simulink model "Janina_hobe_kina_v1"  (R2018a)
settings: Solver=VariableStepAuto  StartTime=0.0  StopTime=0.5  RelTol=1e-3
libraries: fl_lib x37, nesl_utility x19, elec_lib x10, pe_lib x4, powerlib_meascontrol x4
settings Model: Creator=ASUS  LastModifiedBy=ASUS
settings SolverCC: ZeroCrossAlgorithm=Adaptive
settings DebuggingCC: MaxConsecutiveZCsMsg=none

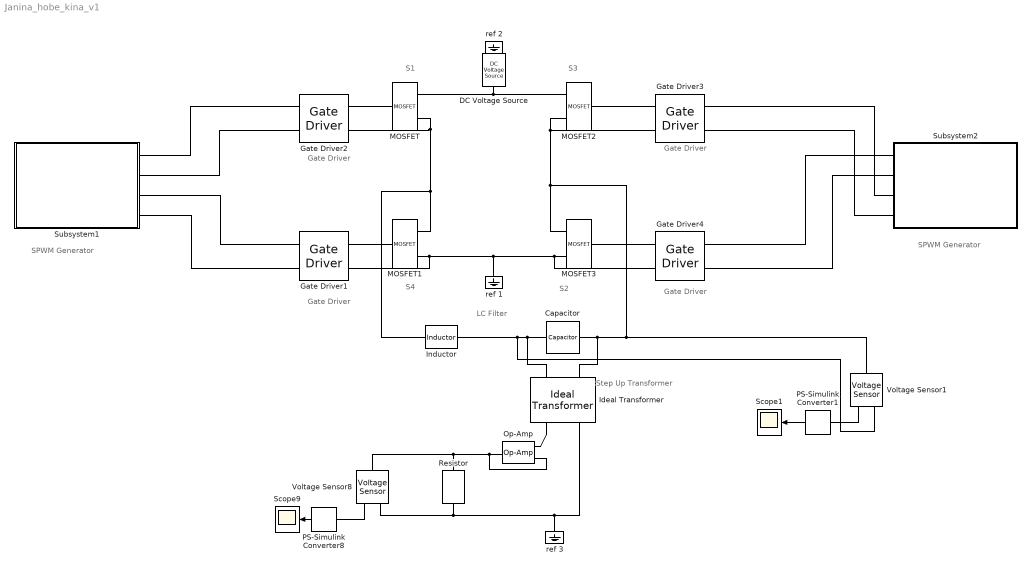
== system Janina_hobe_kina_v1 ==
  note: LC Filter
  note: S1
  note: Gate Driver
  note: SPWM Generator
  note: SPWM Generator
  note: Gate Driver
  note: Gate Driver
  note: Gate Driver
  note: S2
  note: S3
  note: S4
  note: Step Up Transformer
  Capacitor : fl_lib/Electrical/Electrical Elements/Capacitor  c=47e-6 F  r=1e-6 Ohm  g=0 1/Ohm  i_specify=off  i_priority=None  i=0 A  i_nominal_specify=off  i_nominal_unit=A  i_nominal_value=1  v_specify=off  v_priority=None  v=0 V  v_nominal_specify=off  v_nominal_unit=V  v_nominal_value=1  vc_specify=off  vc_priority=High  vc=0 V  vc_nominal_specify=off  vc_nominal_unit=V  vc_nominal_value=1
  DC Voltage Source : fl_lib/Electrical/Electrical Sources/DC Voltage Source  v0=12 V
  Gate Driver{1..4} (4 alike) : elec_lib/Actuators & Drivers/Drivers/Gate Driver  vHigh=15 V  vLow=0 V  parameterization=1  rHigh=2 Ohm  rLow=2 Ohm  tRise=20 ns  tFall=20 ns  cLoad=10 nF  enable_faults=0  t_fault=1 s  fault_type=1  uHighValue=0.7  uLowValue=0.3  tHigh=50 ns  tLow=50 ns  ZonTime_specify=off  ZonTime_priority=None  ZonTime=0 s  ZoffTime_specify=off  ZoffTime_priority=None  ZoffTime=0 s  uHigh=2.0 V  uLow=0.8 V
      settings: SourceProductName=Simscape Electronics  SourceProductBaseCode=SN
  Ideal Transformer : fl_lib/Electrical/Electrical Elements/Ideal Transformer  n=12/220  i1_specify=off  i1_priority=None  i1=0 A  i1_nominal_specify=off  i1_nominal_unit=A  i1_nominal_value=1  v1_specify=off  v1_priority=None  v1=0 V  v1_nominal_specify=off  v1_nominal_unit=V  v1_nominal_value=1  i2_specify=off  i2_priority=None  i2=0 A  i2_nominal_specify=off  i2_nominal_unit=A  i2_nominal_value=1  v2_specify=off  v2_priority=None  v2=0 V  v2_nominal_specify=off  v2_nominal_unit=V  v2_nominal_value=1
      settings: SourceProductName=Simscape  SourceProductBaseCode=SS
  Inductor : elec_lib/Passive Devices/Inductor  l=0.46 H  L_tol=20  enable_L_tol=0  tol_distribution=1  nSigma=4  r=0 Ohm  g=1e-9 1/Ohm  enable_operating_limits=0  operating_limit_action=2  max_working_current=1 A  power_rating=1 W  enable_faults=0  fault_action=1  lambdaPercent=50  k_faulted=0.9999  turnsShort=0  openCct=0  groundShort=0  groundShortG=0 1/Ohm  tau_fault=1e-3 s  enable_temporal_fault=0  t_fault=1 s  enable_behavioral_fault=0  max_permissible_voltage=100 V  n_fail_on_voltage=1  max_permissible_current=1 A  t_fail_on_current=1 s  i_L_specify=off  i_L_priority=High  i_L=0 A  i_L_nominal_specify=off  i_L_nominal_unit=A  i_L_nominal_value=1
      settings: SourceProductName=Simscape Electronics  SourceProductBaseCode=SN
  MOSFET{,1..3} (4 alike) : pe_lib/Semiconductors/Fundamental Components/MOSFET  Rds=0.01 Ohm  Goff=1e-6 1/Ohm  Vth=2 V  diode_param=2  diode_Vf=0.8 V  diode_Ron=0.001 Ohm  diode_Goff=1e-5 1/Ohm  diode_C=5e-8 F  diode_iRM=-235 A  diode_iF=300 A  diode_idot=-50 A/us  diode_trr_param=1  diode_trr_factor=3  diode_trr=15 us  diode_Qrr=1.5e+3 s*uA  thermal_loss_option=2  Voff=300 V  Tau=1e-4 s  Tj=[ 298.15 398.15 ] K  Iout_scalar=600 A  Eon_scalar=0.02286 J  Eoff_scalar=0.01714 J  Von_scalar=2.7 V  Iout_data=[ 0 10 50 100 200 400 600 ] A  Eon_data=[ 0 2.9e-4 0.00143 0.00286 0.00571 0.01314 0.02286; 0 5.7e-4 0.00263 0.00514 0.01029 0.02057 0.03029 ] J  Eoff_data=[ 0 2.1e-4 0.00107 0.00214 0.00429 0.009859999999999999 0.01714; 0 4.3e-4 0.00197 0.00386 0.00771 0.01543 0.02271 ] J  Von_data=[ 0 1.1 1.3 1.45 1.75 2.25 2.7; 0 1 1.15 1.35 1.7 2.35 3 ] V
      settings: SourceProductName=Simscape Power Systems  SourceProductBaseCode=PS
  Op-Amp : fl_lib/Electrical/Electrical Elements/Op-Amp  outI_specify=off  outI_priority=None  outI=0 A  outI_nominal_specify=off  outI_nominal_unit=A  outI_nominal_value=1
  PS-Simulink Converter1 : nesl_utility/PS-Simulink Converter  PhysicalDomain=network_engine_domain  SubClassName=ps_output  LeftPortType=input  RightPortType=output  PseudoPeriodic=off  Frequencies=[]  Unit=1  AffineConversion=off
  PS-Simulink Converter8 : nesl_utility/PS-Simulink Converter  PhysicalDomain=network_engine_domain  SubClassName=ps_output  LeftPortType=input  RightPortType=output  PseudoPeriodic=off  Frequencies=[]  Unit=1  AffineConversion=off
  Resistor : elec_lib/Passive Devices/Resistor  R=100 Ohm  R_tol=5  enable_R_tol=0  tol_distribution=1  nSigma=4  enable_operating_limits=0  operating_limit_action=2  max_working_voltage=100 V  power_rating=1 W  enable_faults=0  fault_action=1  R_faulted=inf Ohm  enable_temporal_fault=0  t_fault=1 s  enable_behavioral_fault=0  max_permissible_current=1 A  t_fail_on_current=1 s  noise_mode=0  sample_time=1e-3 s  repeatability=1  auto_seed=3626636697  user_seed=0  Tdevice=25 degC  alpha=3.93e-3 1/K  Tmeas=25 degC  thermal_mass=100 J/K  power_derating_T1=70 degC  power_derating_T2=155 degC  operating_temperature_range_vec=[-50, 150] degC  temperature_specify=off  temperature_priority=High  temperature=298.15 K  temperature_nominal_specify=off  temperature_nominal_unit=K  temperature_nominal_value=1
  Scope1 : Scope
  Scope9 : Scope
  Subsystem1 : Subsystem
  Subsystem2 : Subsystem
  Voltage Sensor1 : fl_lib/Electrical/Electrical Sensors/Voltage Sensor
  Voltage Sensor8 : fl_lib/Electrical/Electrical Sensors/Voltage Sensor
  ref 1 : fl_lib/Electrical/Electrical Elements/Electrical Reference
  ref 2 : fl_lib/Electrical/Electrical Elements/Electrical Reference
  ref 3 : fl_lib/Electrical/Electrical Elements/Electrical Reference
  wires:
  PS-Simulink Converter8/1 -> Scope9/1
  PS-Simulink Converter1/1 -> Scope1/1
  connections:
  MOSFET/RConn2 -- Gate Driver2/RConn2 -- Inductor/LConn1 -- MOSFET1/RConn1
  ref 2/LConn1 -- DC Voltage Source/RConn1
  MOSFET/RConn1 -- MOSFET2/RConn1 -- DC Voltage Source/LConn1
  MOSFET3/RConn2 -- Gate Driver4/RConn2 -- ref 1/LConn1 -- Gate Driver1/RConn2 -- MOSFET1/RConn2
  Subsystem1/RConn4 -- Gate Driver1/LConn2
  Gate Driver2/LConn1 -- Subsystem1/RConn1
  Gate Driver2/LConn2 -- Subsystem1/RConn2
  Gate Driver1/LConn1 -- Subsystem1/RConn3
  Subsystem2/RConn1 -- Gate Driver4/LConn1
  Subsystem2/RConn2 -- Gate Driver4/LConn2
  Gate Driver3/LConn1 -- Subsystem2/RConn3
  Gate Driver3/LConn2 -- Subsystem2/RConn4
  Gate Driver3/RConn1 -- MOSFET2/LConn1
  Gate Driver4/RConn1 -- MOSFET3/LConn1
  Gate Driver2/RConn1 -- MOSFET/LConn1
  Gate Driver1/RConn1 -- MOSFET1/LConn1
  Capacitor/LConn1 -- Ideal Transformer/LConn1 -- Voltage Sensor1/RConn2 -- Inductor/RConn1
  Op-Amp/LConn1 -- Voltage Sensor8/LConn1 -- Resistor/LConn1 -- Op-Amp/RConn1
  Ideal Transformer/RConn1 -- Op-Amp/LConn2
  Resistor/RConn1 -- ref 3/LConn1 -- Ideal Transformer/RConn2 -- Voltage Sensor8/RConn2
  Voltage Sensor8/RConn1 -- PS-Simulink Converter8/LConn1
  Capacitor/RConn1 -- Voltage Sensor1/LConn1 -- MOSFET3/RConn1 -- Gate Driver3/RConn2 -- MOSFET2/RConn2 -- Ideal Transformer/LConn2
  Voltage Sensor1/RConn1 -- PS-Simulink Converter1/LConn1

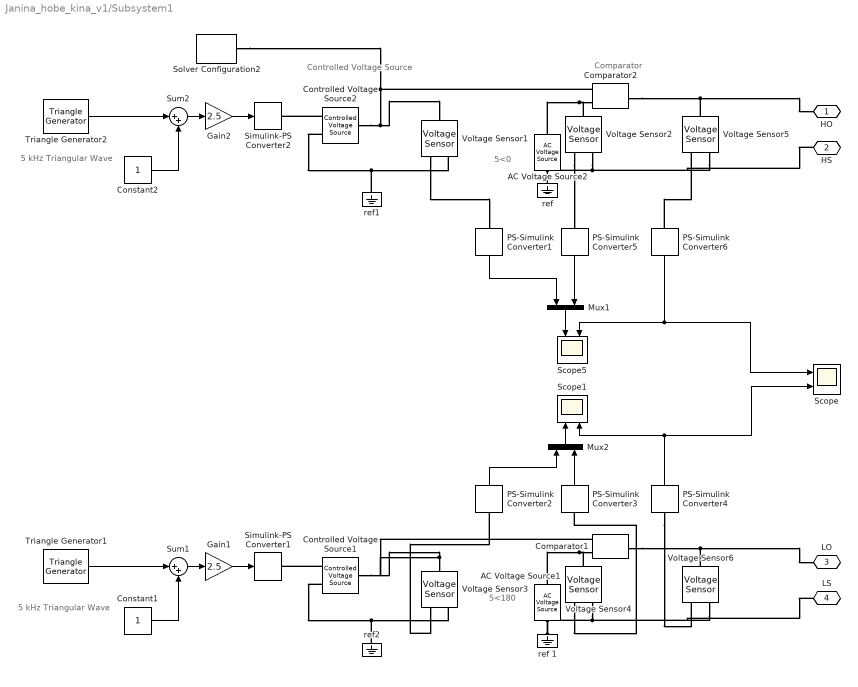
== system Janina_hobe_kina_v1/Subsystem1 ==
  note: Controlled Voltage Source
  note: Comparator
  note: 5 kHz
      | Triangular Wave
  note: 5<180
  note: 5<0
  note: 5 kHz
      | Triangular Wave
  AC Voltage Source1 : fl_lib/Electrical/Electrical Sources/AC Voltage Source  amp=5 V  shift=180 deg  frequency=50 Hz  omega=0 rad/s
  AC Voltage Source2 : fl_lib/Electrical/Electrical Sources/AC Voltage Source  amp=5 V  shift=0 deg  frequency=50 Hz  omega=0 rad/s
  Comparator1 : elec_lib/Integrated Circuits/Comparator  V_OS=5 mV  V_OL=0 V  V_OH=5 V  C_IN=0 pF  R_OUT=50 Ohm  Delay=0 s
      settings: SourceProductName=Simscape Electronics  SourceProductBaseCode=SN
  Comparator2 : elec_lib/Integrated Circuits/Comparator  V_OS=5 mV  V_OL=0 V  V_OH=5 V  C_IN=0 pF  R_OUT=50 Ohm  Delay=0 s
      settings: SourceProductName=Simscape Electronics  SourceProductBaseCode=SN
  Constant1 : Constant
  Constant2 : Constant
  Controlled Voltage Source1 : fl_lib/Electrical/Electrical Sources/Controlled Voltage Source
  Controlled Voltage Source2 : fl_lib/Electrical/Electrical Sources/Controlled Voltage Source
  Gain1 : Gain  Gain=2.5
  Gain2 : Gain  Gain=2.5
  Mux1 : Mux  Inputs=2
  Mux2 : Mux  Inputs=2
  PS-Simulink Converter{1..6} (6 alike) : nesl_utility/PS-Simulink Converter  PhysicalDomain=network_engine_domain  SubClassName=ps_output  LeftPortType=input  RightPortType=output  PseudoPeriodic=off  Frequencies=[]  Unit=1  AffineConversion=off
  Scope : Scope  NumInputPorts=2
  Scope1 : Scope  NumInputPorts=2
  Scope5 : Scope  NumInputPorts=2
  Simulink-PS Converter1 : nesl_utility/Simulink-PS Converter  PhysicalDomain=network_engine_domain  SubClassName=ps_input  LeftPortType=input  RightPortType=output  PseudoPeriodic=off  Frequencies=[]  NoiseDistribution=none  NoiseParameters=[]  Unit=1  AffineConversion=off  FilteringAndDerivatives=provide  SimscapeFilterOrder=1  InputFilterTimeConstant=0.001  UdotUserProvided=0
  Simulink-PS Converter2 : nesl_utility/Simulink-PS Converter  PhysicalDomain=network_engine_domain  SubClassName=ps_input  LeftPortType=input  RightPortType=output  PseudoPeriodic=off  Frequencies=[]  NoiseDistribution=none  NoiseParameters=[]  Unit=1  AffineConversion=off  FilteringAndDerivatives=provide  SimscapeFilterOrder=1  InputFilterTimeConstant=0.001  UdotUserProvided=0
  Solver Configuration2 : nesl_utility/Solver Configuration  PhysicalDomain=network_engine_domain  SubClassName=solver  LeftPortType=input  RightPortType=generic  Tones=[]  Harmonics=[]  SimulateNoise=off  Profile=off  UseLocalSampling=off  EnableSwitchedLinearOptims=on  FrequencyDomain=off  UseCCode=off  RelTol=0.001  AbsTol=1e-06  MinStep=1e-09  ToWorkspace=off  RevertToSquareIcSolve=off  NumHomotopyIterations=100  PhasorMode=off  PhasorModeNumHarmonics=1  DoDC=off  ResidualTolerance=1e-09  UseLocalSolver=off  LocalSolverChoice=NE_BACKWARD_EULER_ADVANCER  LocalSolverSampleTime=0.001  DoFixedCost=off  MaxNonlinIter=3  MaxModeIter=2  LinearAlgebra=Sparse  EquationFormulation=NE_TIME_EF  DelaysMemoryBudget=1024  AutomaticFiltering=on  FilteringTimeConstant=0.001
  Sum1 : Sum  Inputs=|++
  Sum2 : Sum  Inputs=|++
  Triangle Generator1 : powerlib_meascontrol/Pulse & Signal Generators/Triangle Generator  Freq=5e3  Phase=0  Ts=0
  Triangle Generator2 : powerlib_meascontrol/Pulse & Signal Generators/Triangle Generator  Freq=5e3  Phase=0  Ts=0
  Voltage Sensor{1..6} (6 alike) : fl_lib/Electrical/Electrical Sensors/Voltage Sensor
  "ref " : fl_lib/Electrical/Electrical Elements/Electrical Reference
  ref 1 : fl_lib/Electrical/Electrical Elements/Electrical Reference
  ref1 : fl_lib/Electrical/Electrical Elements/Electrical Reference
  ref2 : fl_lib/Electrical/Electrical Elements/Electrical Reference
  HO : PMIOPort  Side=Right
  HS : PMIOPort  Port=2  Side=Right
  LO : PMIOPort  Port=3  Side=Right
  LS : PMIOPort  Port=4  Side=Right
  wires:
  Triangle Generator2/1 -> Sum2/1
  Sum2/1 -> Gain2/1
  Constant2/1 -> Sum2/2
  Gain2/1 -> Simulink-PS Converter2/1
  PS-Simulink Converter5/1 -> Mux1/2
  PS-Simulink Converter1/1 -> Mux1/1
  Mux1/1 -> Scope5/1
  PS-Simulink Converter6/1 -> Scope/1, Scope5/2
  Constant1/1 -> Sum1/2
  Sum1/1 -> Gain1/1
  Gain1/1 -> Simulink-PS Converter1/1
  Triangle Generator1/1 -> Sum1/1
  PS-Simulink Converter2/1 -> Mux2/1
  PS-Simulink Converter3/1 -> Mux2/2
  Mux2/1 -> Scope1/1
  PS-Simulink Converter4/1 -> Scope/2, Scope1/2
  connections:
  Solver Configuration2/RConn1 -- Controlled Voltage Source2/LConn1 -- Voltage Sensor1/LConn1 -- Comparator2/LConn2
  Comparator2/RConn1 -- Voltage Sensor5/LConn1 -- HO/RConn1
  Controlled Voltage Source2/RConn1 -- Simulink-PS Converter2/RConn1
  ref1/LConn1 -- Voltage Sensor1/RConn2 -- Controlled Voltage Source2/RConn2
  Voltage Sensor1/RConn1 -- PS-Simulink Converter1/LConn1
  "ref "/LConn1 -- Voltage Sensor5/RConn2 -- HS/RConn1 -- Voltage Sensor2/RConn2 -- AC Voltage Source2/RConn1
  AC Voltage Source2/LConn1 -- Voltage Sensor2/LConn1 -- Comparator2/LConn1
  Voltage Sensor2/RConn1 -- PS-Simulink Converter5/LConn1
  PS-Simulink Converter6/LConn1 -- Voltage Sensor5/RConn1
  Comparator1/RConn1 -- Voltage Sensor6/LConn1 -- LO/RConn1
  Voltage Sensor3/LConn1 -- Comparator1/LConn2 -- Controlled Voltage Source1/LConn1
  Controlled Voltage Source1/RConn2 -- ref2/LConn1 -- Voltage Sensor3/RConn2
  AC Voltage Source1/RConn1 -- ref 1/LConn1 -- Voltage Sensor6/RConn2 -- LS/RConn1 -- Voltage Sensor4/RConn2
  AC Voltage Source1/LConn1 -- Voltage Sensor4/LConn1 -- Comparator1/LConn1
  Controlled Voltage Source1/RConn1 -- Simulink-PS Converter1/RConn1
  Voltage Sensor3/RConn1 -- PS-Simulink Converter2/LConn1
  PS-Simulink Converter4/LConn1 -- Voltage Sensor6/RConn1
  Voltage Sensor4/RConn1 -- PS-Simulink Converter3/LConn1

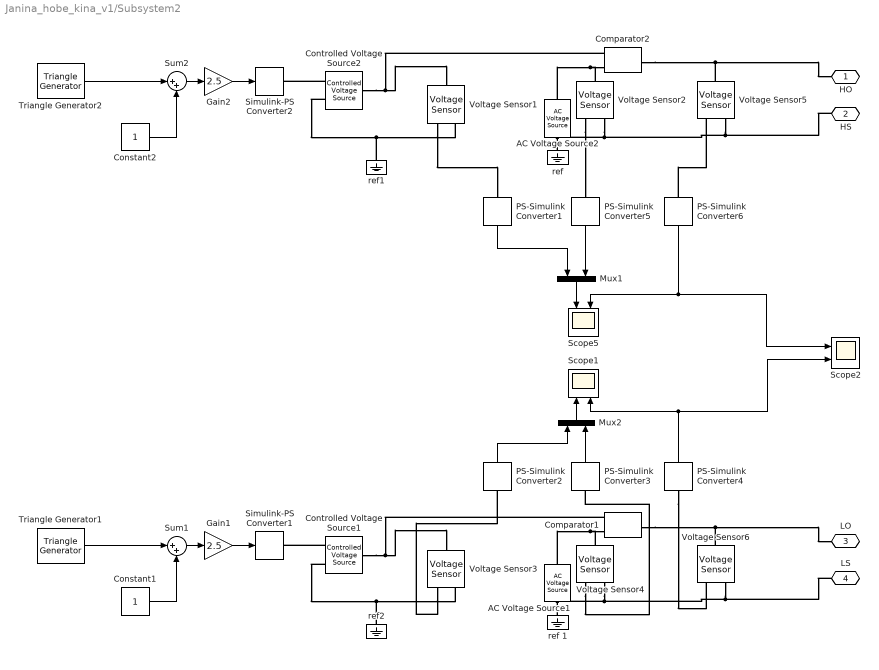
== system Janina_hobe_kina_v1/Subsystem2 ==
  AC Voltage Source1 : fl_lib/Electrical/Electrical Sources/AC Voltage Source  amp=5 V  shift=180 deg  frequency=50 Hz  omega=0 rad/s
  AC Voltage Source2 : fl_lib/Electrical/Electrical Sources/AC Voltage Source  amp=5 V  shift=0 deg  frequency=50 Hz  omega=0 rad/s
  Comparator1 : elec_lib/Integrated Circuits/Comparator  V_OS=5 mV  V_OL=0 V  V_OH=5 V  C_IN=0 pF  R_OUT=50 Ohm  Delay=0 s
      settings: SourceProductName=Simscape Electronics  SourceProductBaseCode=SN
  Comparator2 : elec_lib/Integrated Circuits/Comparator  V_OS=5 mV  V_OL=0 V  V_OH=5 V  C_IN=0 pF  R_OUT=50 Ohm  Delay=0 s
      settings: SourceProductName=Simscape Electronics  SourceProductBaseCode=SN
  Constant1 : Constant
  Constant2 : Constant
  Controlled Voltage Source1 : fl_lib/Electrical/Electrical Sources/Controlled Voltage Source
  Controlled Voltage Source2 : fl_lib/Electrical/Electrical Sources/Controlled Voltage Source
  Gain1 : Gain  Gain=2.5
  Gain2 : Gain  Gain=2.5
  Mux1 : Mux  Inputs=2
  Mux2 : Mux  Inputs=2
  PS-Simulink Converter{1..6} (6 alike) : nesl_utility/PS-Simulink Converter  PhysicalDomain=network_engine_domain  SubClassName=ps_output  LeftPortType=input  RightPortType=output  PseudoPeriodic=off  Frequencies=[]  Unit=1  AffineConversion=off
  Scope1 : Scope  NumInputPorts=2
  Scope2 : Scope  NumInputPorts=2
  Scope5 : Scope  NumInputPorts=2
  Simulink-PS Converter1 : nesl_utility/Simulink-PS Converter  PhysicalDomain=network_engine_domain  SubClassName=ps_input  LeftPortType=input  RightPortType=output  PseudoPeriodic=off  Frequencies=[]  NoiseDistribution=none  NoiseParameters=[]  Unit=1  AffineConversion=off  FilteringAndDerivatives=provide  SimscapeFilterOrder=1  InputFilterTimeConstant=0.001  UdotUserProvided=0
  Simulink-PS Converter2 : nesl_utility/Simulink-PS Converter  PhysicalDomain=network_engine_domain  SubClassName=ps_input  LeftPortType=input  RightPortType=output  PseudoPeriodic=off  Frequencies=[]  NoiseDistribution=none  NoiseParameters=[]  Unit=1  AffineConversion=off  FilteringAndDerivatives=provide  SimscapeFilterOrder=1  InputFilterTimeConstant=0.001  UdotUserProvided=0
  Sum1 : Sum  Inputs=|++
  Sum2 : Sum  Inputs=|++
  Triangle Generator1 : powerlib_meascontrol/Pulse & Signal Generators/Triangle Generator  Freq=5e3  Phase=0  Ts=0
  Triangle Generator2 : powerlib_meascontrol/Pulse & Signal Generators/Triangle Generator  Freq=5e3  Phase=0  Ts=0
  Voltage Sensor{1..6} (6 alike) : fl_lib/Electrical/Electrical Sensors/Voltage Sensor
  "ref " : fl_lib/Electrical/Electrical Elements/Electrical Reference
  ref 1 : fl_lib/Electrical/Electrical Elements/Electrical Reference
  ref1 : fl_lib/Electrical/Electrical Elements/Electrical Reference
  ref2 : fl_lib/Electrical/Electrical Elements/Electrical Reference
  HO : PMIOPort  Side=Right
  HS : PMIOPort  Port=2  Side=Right
  LO : PMIOPort  Port=3  Side=Right
  LS : PMIOPort  Port=4  Side=Right
  wires:
  Triangle Generator2/1 -> Sum2/1
  Sum2/1 -> Gain2/1
  Constant2/1 -> Sum2/2
  Gain2/1 -> Simulink-PS Converter2/1
  PS-Simulink Converter5/1 -> Mux1/2
  PS-Simulink Converter1/1 -> Mux1/1
  Mux1/1 -> Scope5/1
  PS-Simulink Converter6/1 -> Scope2/1, Scope5/2
  Constant1/1 -> Sum1/2
  Sum1/1 -> Gain1/1
  Gain1/1 -> Simulink-PS Converter1/1
  Triangle Generator1/1 -> Sum1/1
  PS-Simulink Converter2/1 -> Mux2/1
  PS-Simulink Converter3/1 -> Mux2/2
  Mux2/1 -> Scope1/1
  PS-Simulink Converter4/1 -> Scope2/2, Scope1/2
  connections:
  Controlled Voltage Source2/LConn1 -- Comparator2/LConn2 -- Voltage Sensor1/LConn1
  HO/RConn1 -- Comparator2/RConn1 -- Voltage Sensor5/LConn1
  Controlled Voltage Source2/RConn1 -- Simulink-PS Converter2/RConn1
  ref1/LConn1 -- Voltage Sensor1/RConn2 -- Controlled Voltage Source2/RConn2
  Voltage Sensor1/RConn1 -- PS-Simulink Converter1/LConn1
  Voltage Sensor2/RConn2 -- "ref "/LConn1 -- AC Voltage Source2/RConn1 -- HS/RConn1 -- Voltage Sensor5/RConn2
  Comparator2/LConn1 -- AC Voltage Source2/LConn1 -- Voltage Sensor2/LConn1
  Voltage Sensor2/RConn1 -- PS-Simulink Converter5/LConn1
  PS-Simulink Converter6/LConn1 -- Voltage Sensor5/RConn1
  Comparator1/RConn1 -- LO/RConn1 -- Voltage Sensor6/LConn1
  Controlled Voltage Source1/LConn1 -- Voltage Sensor3/LConn1 -- Comparator1/LConn2
  Controlled Voltage Source1/RConn2 -- Voltage Sensor3/RConn2 -- ref2/LConn1
  Voltage Sensor4/RConn2 -- ref 1/LConn1 -- AC Voltage Source1/RConn1 -- Voltage Sensor6/RConn2 -- LS/RConn1
  AC Voltage Source1/LConn1 -- Comparator1/LConn1 -- Voltage Sensor4/LConn1
  Controlled Voltage Source1/RConn1 -- Simulink-PS Converter1/RConn1
  Voltage Sensor3/RConn1 -- PS-Simulink Converter2/LConn1
  PS-Simulink Converter4/LConn1 -- Voltage Sensor6/RConn1
  Voltage Sensor4/RConn1 -- PS-Simulink Converter3/LConn1
